simulink model "Simulacao_POSITIVO_LQG"  (R2020a)
settings: Solver=VariableStepAuto  StartTime=0.0  StopTime=15  RelTol=1e-6
values from neighbouring files (symbols this model uses):
  K1_rd1 = Kchz1(1,1)    [LQG_DIRSCRETO_1406_2025_NEGATIVO.m]    (also in LQG_DIRSCRETO_1406_2025_POSITIVO.m)
  K1_rd2 = Kchz2(1,1)    [LQG_DIRSCRETO_1406_2025_NEGATIVO.m]    (also in LQG_DIRSCRETO_1406_2025_POSITIVO.m)
  K1_rd3 = Kchz3(1,1)    [LQG_DIRSCRETO_1406_2025_NEGATIVO.m]    (also in LQG_DIRSCRETO_1406_2025_POSITIVO.m)
  K1_re1 = Kchz1(1,1)    [LQG_DIRSCRETO_1406_2025_NEGATIVO.m]    (also in LQG_DIRSCRETO_1406_2025_POSITIVO.m)
  K1_re2 = Kchz2(1,1)    [LQG_DIRSCRETO_1406_2025_NEGATIVO.m]    (also in LQG_DIRSCRETO_1406_2025_POSITIVO.m)
  K1_re3 = Kchz3(1,1)    [LQG_DIRSCRETO_1406_2025_NEGATIVO.m]    (also in LQG_DIRSCRETO_1406_2025_POSITIVO.m)
  Ki_rd1 = -Kchz1(1,2)    [LQG_DIRSCRETO_1406_2025_NEGATIVO.m]    (also in LQG_DIRSCRETO_1406_2025_POSITIVO.m)
  Ki_rd2 = -Kchz2(1,2)    [LQG_DIRSCRETO_1406_2025_NEGATIVO.m]    (also in LQG_DIRSCRETO_1406_2025_POSITIVO.m)
  Ki_rd3 = -Kchz3(1,2)    [LQG_DIRSCRETO_1406_2025_NEGATIVO.m]    (also in LQG_DIRSCRETO_1406_2025_POSITIVO.m)
  Ki_re1 = -Kchz1(1,2)    [LQG_DIRSCRETO_1406_2025_NEGATIVO.m]    (also in LQG_DIRSCRETO_1406_2025_POSITIVO.m)
  Ki_re2 = -Kchz2(1,2)    [LQG_DIRSCRETO_1406_2025_NEGATIVO.m]    (also in LQG_DIRSCRETO_1406_2025_POSITIVO.m)
  Ki_re3 = -Kchz3(1,2)    [LQG_DIRSCRETO_1406_2025_NEGATIVO.m]    (also in LQG_DIRSCRETO_1406_2025_POSITIVO.m)
  Ts = 0.02    [LQG_DIRSCRETO_1406_2025_NEGATIVO.m]    (also in LQG_DIRSCRETO_1406_2025_POSITIVO.m)
undefined symbols (not defined in the file or in its folder): A_rd1, A_rd2, A_rd3, A_re1, A_re2, A_re3, B_rd1, B_rd2, B_rd3, B_re1, B_re2, B_re3, C_rd1, C_rd2, C_rd3, C_re1, C_re2, C_re3, DiscIntNeverNeededParam, Ke_rd1, Ke_rd2, Ke_rd3, Ke_re1, Ke_re2, Ke_re3, sigbuilder_block
settings Model: Creator=vinic  LastModifiedBy=vinic

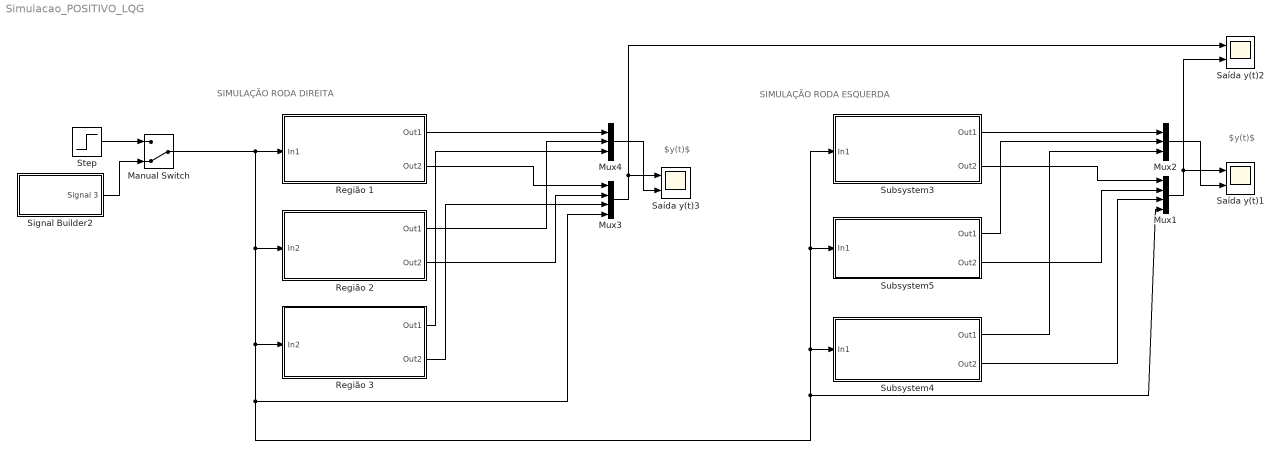
== system Simulacao_POSITIVO_LQG ==
  note: SIMULAÇÃO RODA ESQUERDA
  note: SIMULAÇÃO RODA DIREITA
  note: $y(t)$
  note: $y(t)$
  Manual Switch : ManualSwitch  CurrentSetting=0
  Mux1 : Mux
  Mux2 : Mux  Inputs=3
  Mux3 : Mux
  Mux4 : Mux  Inputs=3
  Região 1 : Subsystem
  Região 2 : Subsystem
  Região 3 : Subsystem
  Saída y(t)1 : Scope  NumInputPorts=2
  Saída y(t)2 : Scope  NumInputPorts=2
  Saída y(t)3 : Scope  NumInputPorts=2
  Signal Builder2 : Subsystem  Tag=STV Subsys  LoadFcn=sigbuilder_block('load');  StartFcn=sigbuilder_block('start');  StopFcn=sigbuilder_block('stop');  ClipboardFcn=sigbuilder_block('clipboard');  mask(Sigbuilder block){tuvar=[0:10]}
      mask help: Simulink:masks:SigbuilderBlock_MD
      mask init:
      | if ~strcmp(get_param(bdroot(gcbh),'SimulationStatus'),'stopped') tuvar = sigbuilder_block('maskInit'); end
      settings: CopyFcn=sigbuilder_block('copy');  DeleteFcn=sigbuilder_block('delete');  ModelCloseFcn=sigbuilder_block('modelClose');  PreSaveFcn=sigbuilder_block('preSave');  PauseFcn=sigbuilder_block('pause');  ContinueFcn=sigbuilder_block('continue');  NameChangeFcn=sigbuilder_block('namechange');  OpenFcn=sigbuilder_block('open',[5.4 36 1141.2 516.6 ]);  CloseFcn=sigbuilder_block('close');
      mask Display: plot(0, 0, 100, 100,[2, 2, 32, 32, 2], [68, 8, 8, 68, 68],[32, 2], [38, 38], [32, 19, 2],[53, 60, 44], [32, 17, 17, 2],[16, 16, 31, 31]);txt = getActiveGroup(gcbh);text(2, 100, txt,'verticalAlignment', 'top');
  Step : Step  Time=0  After=500  SampleTime=0.02
  Subsystem3 : Subsystem
  Subsystem4 : Subsystem
  Subsystem5 : Subsystem
  wires:
  Mux4/1 -> Saída y(t)3/2
  Step/1 -> Manual Switch/1
  Região 1/1(Out1) -> Mux4/1
  Região 2/1(Out1) -> Mux4/2
  Região 2/2(Out2) -> Mux3/2
  Região 3/1(Out1) -> Mux4/3
  Região 3/2(Out2) -> Mux3/3
  Mux3/1 -> Saída y(t)3/1, Saída y(t)2/1
  Região 1/2(Out2) -> Mux3/1
  Mux2/1 -> Saída y(t)1/2
  Subsystem5/2(Out2) -> Mux1/2
  Subsystem3/2(Out2) -> Mux1/1
  Subsystem5/1(Out1) -> Mux2/2
  Subsystem4/1(Out1) -> Mux2/3
  Mux1/1 -> Saída y(t)2/2, Saída y(t)1/1
  Subsystem4/2(Out2) -> Mux1/3
  Manual Switch/1 -> Região 3/1(In2), Mux3/4, Subsystem4/1(In1), Subsystem3/1(In1), Subsystem5/1(In1), Mux1/4, Região 2/1(In2), Região 1/1(In1)
  Subsystem3/1(Out1) -> Mux2/1
  Signal Builder2/1(Signal 3) -> Manual Switch/2

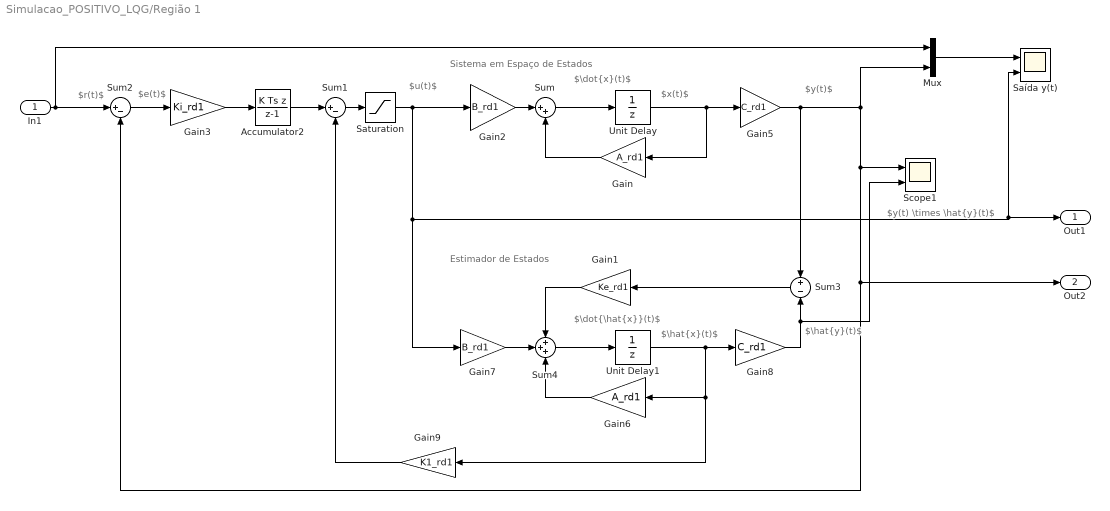
== system Simulacao_POSITIVO_LQG/Região 1 ==
  note: $\hat{y}(t)$
  note: Estimador de Estados
  note: $e(t)$
  note: $\dot{x}(t)$
  note: $\hat{x}(t)$
  note: $y(t)$
  note: $\dot{\hat{x}}(t)$
  note: $u(t)$
  note: $r(t)$
  note: $y(t) \times \hat{y}(t)$
  note: $x(t)$
  note: Sistema em Espaço de Estados
  In1 : Inport
  Accumulator2 : DiscreteIntegrator  IntegratorMethod=Integration: Backward Euler  SampleTime=Ts  ICPrevOutput=DiscIntNeverNeededParam  ICPrevScaledInput=DiscIntNeverNeededParam
  Gain : Gain  Gain=A_rd1
  Gain1 : Gain  Gain=Ke_rd1
  Gain2 : Gain  Gain=B_rd1
  Gain3 : Gain  Gain=Ki_rd1
  Gain5 : Gain  Gain=C_rd1
  Gain6 : Gain  Gain=A_rd1
  Gain7 : Gain  Gain=B_rd1
  Gain8 : Gain  Gain=C_rd1
  Gain9 : Gain  Gain=K1_rd1
  Mux : Mux  Inputs=2
  Saturation : Saturate  UpperLimit=100  LowerLimit=-100
  Saída y(t) : Scope  NumInputPorts=2
  Scope1 : Scope  NumInputPorts=2
  Sum : Sum  Inputs=|++
  Sum1 : Sum  Inputs=|+-
  Sum2 : Sum  Inputs=|+-
  Sum3 : Sum  Inputs=+|-
  Sum4 : Sum  Inputs=+++
  Unit Delay : UnitDelay  SampleTime=Ts  HasFrameUpgradeWarning=on
  Unit Delay1 : UnitDelay  SampleTime=Ts  HasFrameUpgradeWarning=on
  Out1 : Outport
  Out2 : Outport  Port=2
  wires:
  Mux/1 -> Saída y(t)/1
  Gain1/1 -> Sum4/1
  Gain6/1 -> Sum4/3
  Gain3/1 -> Accumulator2/1
  Saturation/1 -> Gain7/1, Out1/1, Saída y(t)/2, Gain2/1
  Sum1/1 -> Saturation/1
  Sum4/1 -> Unit Delay1/1
  Gain8/1 -> Scope1/2, Sum3/2
  Gain/1 -> Sum/2
  Unit Delay1/1 -> Gain9/1, Gain6/1, Gain8/1
  Gain5/1 -> Sum3/1, Scope1/1, Sum2/2, Out2/1, Mux/2
  Unit Delay/1 -> Gain5/1, Gain/1
  Gain9/1 -> Sum1/2
  Gain2/1 -> Sum/1
  Gain7/1 -> Sum4/2
  Sum2/1 -> Gain3/1
  Accumulator2/1 -> Sum1/1
  In1/1 -> Mux/1, Sum2/1
  Sum3/1 -> Gain1/1
  Sum/1 -> Unit Delay/1

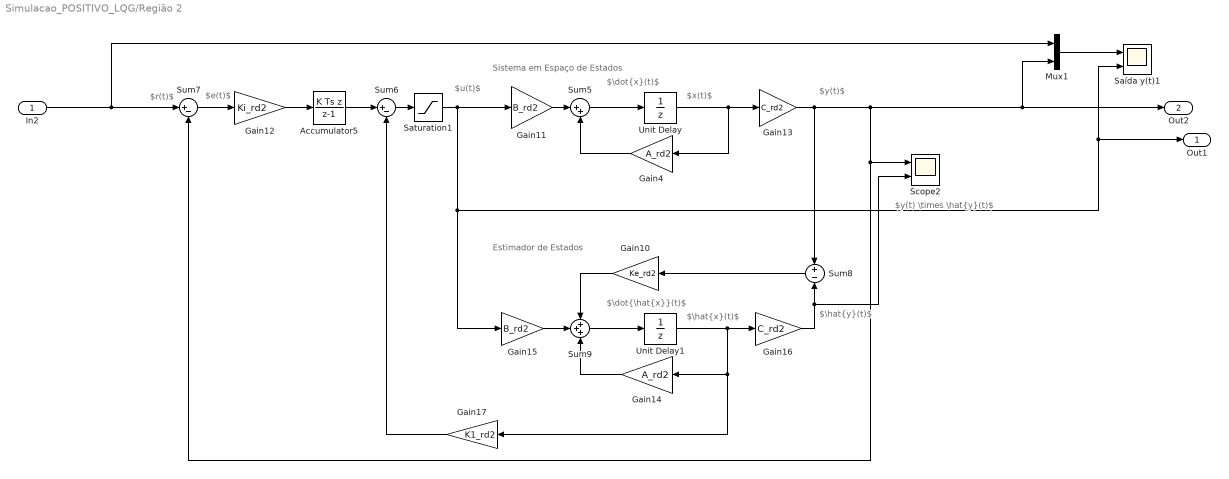
== system Simulacao_POSITIVO_LQG/Região 2 ==
  note: $r(t)$
  note: Sistema em Espaço de Estados
  note: $e(t)$
  note: $\dot{\hat{x}}(t)$
  note: $\hat{x}(t)$
  note: Estimador de Estados
  note: $x(t)$
  note: $u(t)$
  note: $y(t) \times \hat{y}(t)$
  note: $y(t)$
  note: $\hat{y}(t)$
  note: $\dot{x}(t)$
  In2 : Inport
  Accumulator5 : DiscreteIntegrator  IntegratorMethod=Integration: Backward Euler  SampleTime=Ts  ICPrevOutput=DiscIntNeverNeededParam  ICPrevScaledInput=DiscIntNeverNeededParam
  Gain10 : Gain  Gain=Ke_rd2
  Gain11 : Gain  Gain=B_rd2
  Gain12 : Gain  Gain=Ki_rd2
  Gain13 : Gain  Gain=C_rd2
  Gain14 : Gain  Gain=A_rd2
  Gain15 : Gain  Gain=B_rd2
  Gain16 : Gain  Gain=C_rd2
  Gain17 : Gain  Gain=K1_rd2
  Gain4 : Gain  Gain=A_rd2
  Mux1 : Mux  Inputs=2
  Saturation1 : Saturate  UpperLimit=100  LowerLimit=-100
  Saída y(t)1 : Scope  NumInputPorts=2
  Scope2 : Scope  NumInputPorts=2
  Sum5 : Sum  Inputs=|++
  Sum6 : Sum  Inputs=|+-
  Sum7 : Sum  Inputs=|+-
  Sum8 : Sum  Inputs=+|-
  Sum9 : Sum  Inputs=+++
  Unit Delay : UnitDelay  SampleTime=-1  HasFrameUpgradeWarning=on
  Unit Delay1 : UnitDelay  SampleTime=-1  HasFrameUpgradeWarning=on
  Out1 : Outport
  Out2 : Outport  Port=2
  wires:
  Gain13/1 -> Sum8/1, Mux1/2, Out2/1, Scope2/1, Sum7/2
  Gain10/1 -> Sum9/1
  Mux1/1 -> Saída y(t)1/1
  Unit Delay1/1 -> Gain17/1, Gain14/1, Gain16/1
  Sum9/1 -> Unit Delay1/1
  Gain15/1 -> Sum9/2
  Unit Delay/1 -> Gain13/1, Gain4/1
  Saturation1/1 -> Out1/1, Saída y(t)1/2, Gain15/1, Gain11/1
  Gain11/1 -> Sum5/1
  Gain17/1 -> Sum6/2
  Sum6/1 -> Saturation1/1
  Sum5/1 -> Unit Delay/1
  Gain16/1 -> Scope2/2, Sum8/2
  Accumulator5/1 -> Sum6/1
  Gain4/1 -> Sum5/2
  Gain12/1 -> Accumulator5/1
  Sum7/1 -> Gain12/1
  Gain14/1 -> Sum9/3
  In2/1 -> Mux1/1, Sum7/1
  Sum8/1 -> Gain10/1

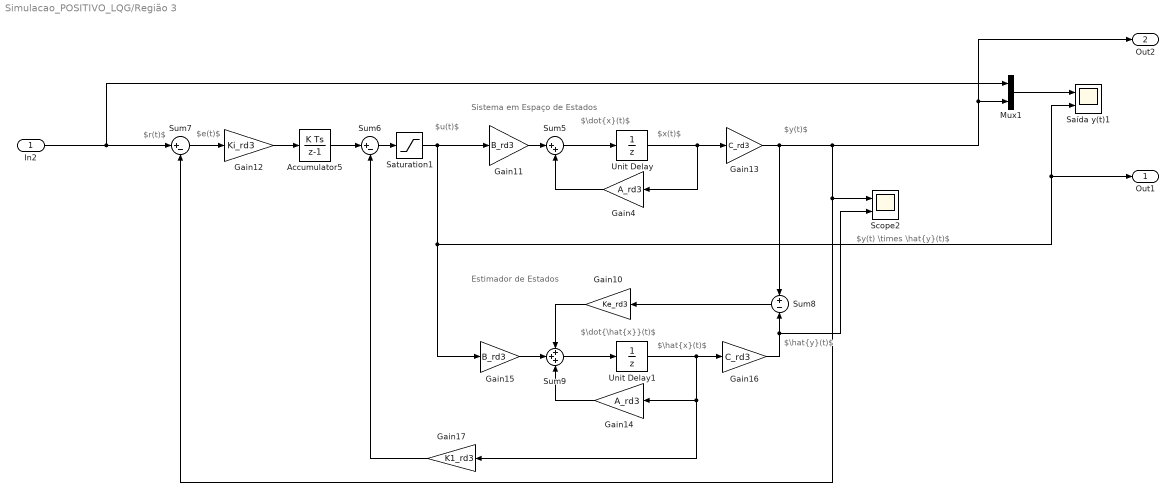
== system Simulacao_POSITIVO_LQG/Região 3 ==
  note: $\dot{\hat{x}}(t)$
  note: Estimador de Estados
  note: $y(t)$
  note: Sistema em Espaço de Estados
  note: $u(t)$
  note: $x(t)$
  note: $r(t)$
  note: $y(t) \times \hat{y}(t)$
  note: $e(t)$
  note: $\hat{y}(t)$
  note: $\dot{x}(t)$
  note: $\hat{x}(t)$
  In2 : Inport
  Accumulator5 : DiscreteIntegrator  SampleTime=Ts  ICPrevOutput=DiscIntNeverNeededParam  ICPrevScaledInput=DiscIntNeverNeededParam
  Gain10 : Gain  Gain=Ke_rd3
  Gain11 : Gain  Gain=B_rd3
  Gain12 : Gain  Gain=Ki_rd3
  Gain13 : Gain  Gain=C_rd3
  Gain14 : Gain  Gain=A_rd3
  Gain15 : Gain  Gain=B_rd3
  Gain16 : Gain  Gain=C_rd3
  Gain17 : Gain  Gain=K1_rd3
  Gain4 : Gain  Gain=A_rd3
  Mux1 : Mux  Inputs=2
  Saturation1 : Saturate  UpperLimit=100  LowerLimit=-100
  Saída y(t)1 : Scope  NumInputPorts=2
  Scope2 : Scope  NumInputPorts=2
  Sum5 : Sum  Inputs=|++
  Sum6 : Sum  Inputs=|+-
  Sum7 : Sum  Inputs=|+-
  Sum8 : Sum  Inputs=+|-
  Sum9 : Sum  Inputs=+++
  Unit Delay : UnitDelay  SampleTime=Ts  HasFrameUpgradeWarning=on
  Unit Delay1 : UnitDelay  SampleTime=Ts  HasFrameUpgradeWarning=on
  Out1 : Outport
  Out2 : Outport  Port=2
  wires:
  Unit Delay/1 -> Gain13/1, Gain4/1
  In2/1 -> Mux1/1, Sum7/1
  Gain14/1 -> Sum9/3
  Gain11/1 -> Sum5/1
  Gain12/1 -> Accumulator5/1
  Accumulator5/1 -> Sum6/1
  Sum7/1 -> Gain12/1
  Gain16/1 -> Scope2/2, Sum8/2
  Gain17/1 -> Sum6/2
  Saturation1/1 -> Out1/1, Saída y(t)1/2, Gain15/1, Gain11/1
  Unit Delay1/1 -> Gain17/1, Gain14/1, Gain16/1
  Gain15/1 -> Sum9/2
  Sum6/1 -> Saturation1/1
  Gain4/1 -> Sum5/2
  Gain13/1 -> Sum8/1, Mux1/2, Out2/1, Scope2/1, Sum7/2
  Sum5/1 -> Unit Delay/1
  Mux1/1 -> Saída y(t)1/1
  Gain10/1 -> Sum9/1
  Sum9/1 -> Unit Delay1/1
  Sum8/1 -> Gain10/1

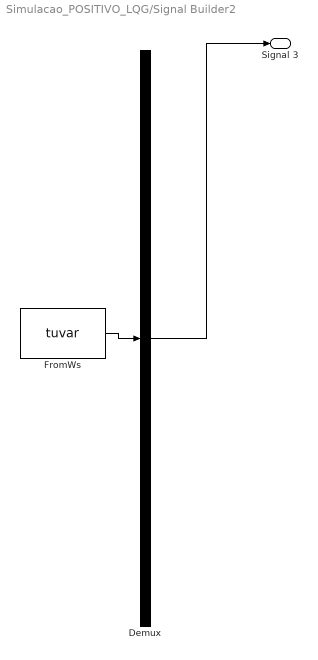
== system Simulacao_POSITIVO_LQG/Signal Builder2 ==
  Demux : Demux  Tag=STV Demux  Outputs=1
      settings: DisplayOption=none
  FromWs : FromWorkspace  Tag=STV FromWs  VariableName=tuvar
      SigBuilderData=|
      | common.afterFinalStr = 'Extrapolate'
      | common.sampleTime = 0
      | dataSet.timeRange = [0 15]
      | dataSet.name = 'Group 1'
      | sbobj.Groups.Name = 'Group 1'
      | sbobj.Groups.Signals.Name = 'Signal 3'
      | sbobj.Groups.Signals.XData = [0 2.5 2.5 5 5 7.5 7.5 10 10 12.5 12.5 15]
      | sbobj.Groups.Signals.YData = [320 320 560 560 800 800 400 400 640 640 480 480]
      | sbobj.Groups.TimeRange = [0 15]
  Signal 3 : Outport  Tag=STV Outport
  wires:
  FromWs/1 -> Demux/1
  Demux/1 -> Signal 3/1

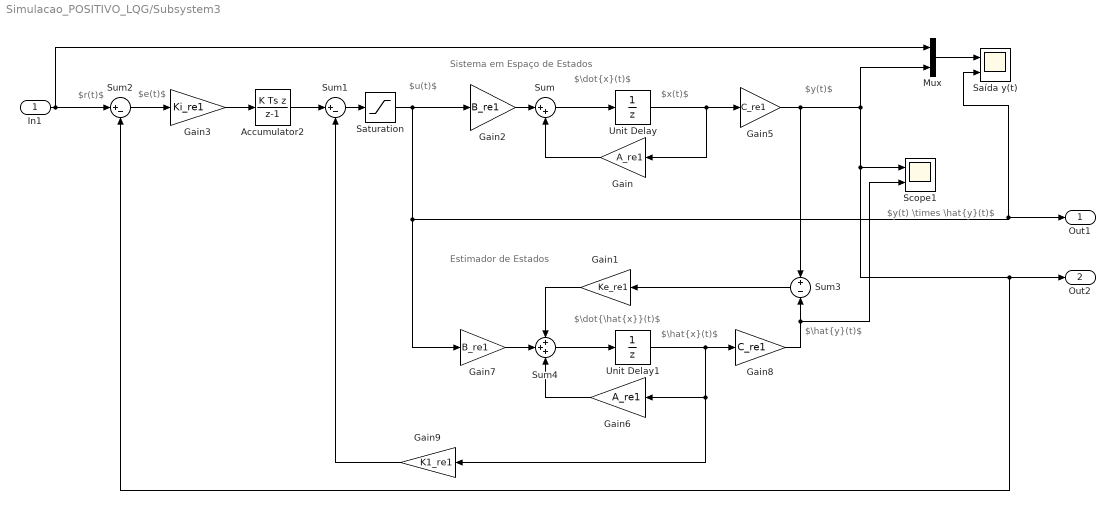
== system Simulacao_POSITIVO_LQG/Subsystem3 ==
  note: $\hat{y}(t)$
  note: Estimador de Estados
  note: $e(t)$
  note: $\dot{x}(t)$
  note: $\hat{x}(t)$
  note: $y(t)$
  note: $\dot{\hat{x}}(t)$
  note: $u(t)$
  note: $r(t)$
  note: $y(t) \times \hat{y}(t)$
  note: $x(t)$
  note: Sistema em Espaço de Estados
  In1 : Inport
  Accumulator2 : DiscreteIntegrator  IntegratorMethod=Integration: Backward Euler  SampleTime=Ts  ICPrevOutput=DiscIntNeverNeededParam  ICPrevScaledInput=DiscIntNeverNeededParam
  Gain : Gain  Gain=A_re1
  Gain1 : Gain  Gain=Ke_re1
  Gain2 : Gain  Gain=B_re1
  Gain3 : Gain  Gain=Ki_re1
  Gain5 : Gain  Gain=C_re1
  Gain6 : Gain  Gain=A_re1
  Gain7 : Gain  Gain=B_re1
  Gain8 : Gain  Gain=C_re1
  Gain9 : Gain  Gain=K1_re1
  Mux : Mux  Inputs=2
  Saturation : Saturate  UpperLimit=100  LowerLimit=-100
  Saída y(t) : Scope  NumInputPorts=2
  Scope1 : Scope  NumInputPorts=2
  Sum : Sum  Inputs=|++
  Sum1 : Sum  Inputs=|+-
  Sum2 : Sum  Inputs=|+-
  Sum3 : Sum  Inputs=+|-
  Sum4 : Sum  Inputs=+++
  Unit Delay : UnitDelay  SampleTime=Ts  HasFrameUpgradeWarning=on
  Unit Delay1 : UnitDelay  SampleTime=Ts  HasFrameUpgradeWarning=on
  Out1 : Outport
  Out2 : Outport  Port=2
  wires:
  Mux/1 -> Saída y(t)/1
  Gain1/1 -> Sum4/1
  Gain6/1 -> Sum4/3
  Gain3/1 -> Accumulator2/1
  Saturation/1 -> Gain7/1, Out1/1, Saída y(t)/2, Gain2/1
  Sum1/1 -> Saturation/1
  Sum4/1 -> Unit Delay1/1
  Gain8/1 -> Scope1/2, Sum3/2
  Gain/1 -> Sum/2
  Unit Delay1/1 -> Gain9/1, Gain6/1, Gain8/1
  Gain5/1 -> Sum3/1, Scope1/1, Sum2/2, Out2/1, Mux/2
  Unit Delay/1 -> Gain5/1, Gain/1
  Gain9/1 -> Sum1/2
  Gain2/1 -> Sum/1
  Gain7/1 -> Sum4/2
  Sum2/1 -> Gain3/1
  Accumulator2/1 -> Sum1/1
  In1/1 -> Mux/1, Sum2/1
  Sum3/1 -> Gain1/1
  Sum/1 -> Unit Delay/1

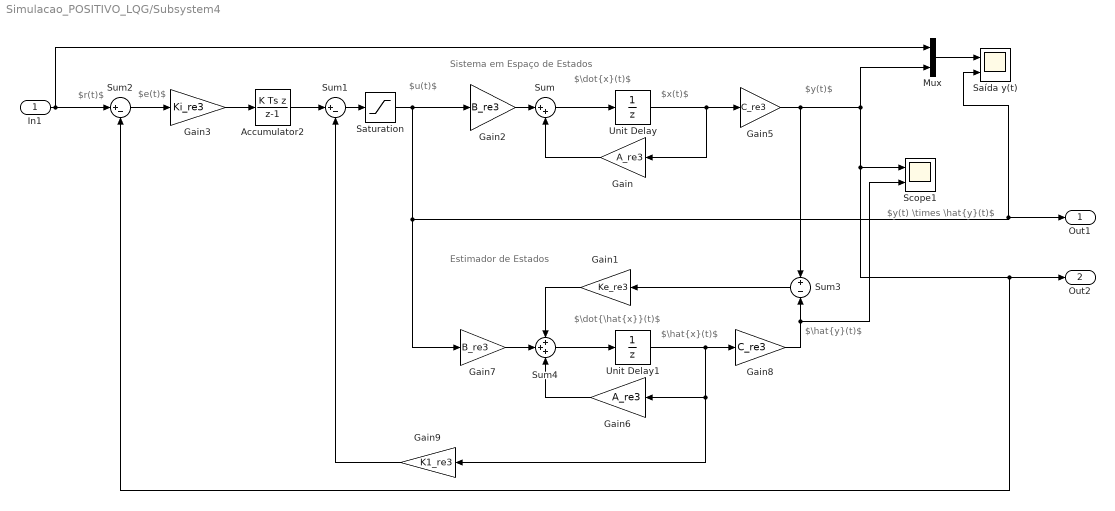
== system Simulacao_POSITIVO_LQG/Subsystem4 ==
  note: Estimador de Estados
  note: $e(t)$
  note: $\hat{y}(t)$
  note: $\dot{x}(t)$
  note: $y(t)$
  note: $u(t)$
  note: $r(t)$
  note: $\dot{\hat{x}}(t)$
  note: $x(t)$
  note: $y(t) \times \hat{y}(t)$
  note: $\hat{x}(t)$
  note: Sistema em Espaço de Estados
  In1 : Inport
  Accumulator2 : DiscreteIntegrator  IntegratorMethod=Integration: Backward Euler  SampleTime=Ts  ICPrevOutput=DiscIntNeverNeededParam  ICPrevScaledInput=DiscIntNeverNeededParam
  Gain : Gain  Gain=A_re3
  Gain1 : Gain  Gain=Ke_re3
  Gain2 : Gain  Gain=B_re3
  Gain3 : Gain  Gain=Ki_re3
  Gain5 : Gain  Gain=C_re3
  Gain6 : Gain  Gain=A_re3
  Gain7 : Gain  Gain=B_re3
  Gain8 : Gain  Gain=C_re3
  Gain9 : Gain  Gain=K1_re3
  Mux : Mux  Inputs=2
  Saturation : Saturate  UpperLimit=100  LowerLimit=-100
  Saída y(t) : Scope  NumInputPorts=2
  Scope1 : Scope  NumInputPorts=2
  Sum : Sum  Inputs=|++
  Sum1 : Sum  Inputs=|+-
  Sum2 : Sum  Inputs=|+-
  Sum3 : Sum  Inputs=+|-
  Sum4 : Sum  Inputs=+++
  Unit Delay : UnitDelay  SampleTime=Ts  HasFrameUpgradeWarning=on
  Unit Delay1 : UnitDelay  SampleTime=Ts  HasFrameUpgradeWarning=on
  Out1 : Outport
  Out2 : Outport  Port=2
  wires:
  Sum/1 -> Unit Delay/1
  Sum2/1 -> Gain3/1
  Sum3/1 -> Gain1/1
  Gain5/1 -> Sum3/1, Scope1/1, Sum2/2, Out2/1, Mux/2
  Accumulator2/1 -> Sum1/1
  Gain/1 -> Sum/2
  In1/1 -> Mux/1, Sum2/1
  Gain8/1 -> Scope1/2, Sum3/2
  Unit Delay1/1 -> Gain9/1, Gain6/1, Gain8/1
  Gain9/1 -> Sum1/2
  Gain1/1 -> Sum4/1
  Gain3/1 -> Accumulator2/1
  Gain2/1 -> Sum/1
  Saturation/1 -> Gain7/1, Out1/1, Saída y(t)/2, Gain2/1
  Gain7/1 -> Sum4/2
  Mux/1 -> Saída y(t)/1
  Sum1/1 -> Saturation/1
  Sum4/1 -> Unit Delay1/1
  Gain6/1 -> Sum4/3
  Unit Delay/1 -> Gain5/1, Gain/1

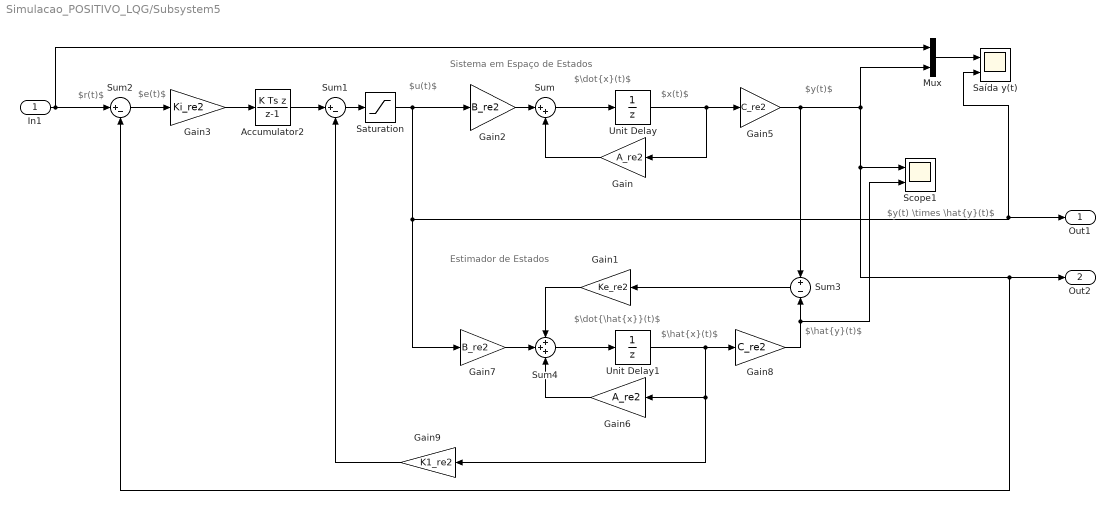
== system Simulacao_POSITIVO_LQG/Subsystem5 ==
  note: Estimador de Estados
  note: $e(t)$
  note: $\hat{y}(t)$
  note: $\dot{x}(t)$
  note: $y(t)$
  note: $u(t)$
  note: $r(t)$
  note: $\dot{\hat{x}}(t)$
  note: $x(t)$
  note: $y(t) \times \hat{y}(t)$
  note: $\hat{x}(t)$
  note: Sistema em Espaço de Estados
  In1 : Inport
  Accumulator2 : DiscreteIntegrator  IntegratorMethod=Integration: Backward Euler  SampleTime=Ts  ICPrevOutput=DiscIntNeverNeededParam  ICPrevScaledInput=DiscIntNeverNeededParam
  Gain : Gain  Gain=A_re2
  Gain1 : Gain  Gain=Ke_re2
  Gain2 : Gain  Gain=B_re2
  Gain3 : Gain  Gain=Ki_re2
  Gain5 : Gain  Gain=C_re2
  Gain6 : Gain  Gain=A_re2
  Gain7 : Gain  Gain=B_re2
  Gain8 : Gain  Gain=C_re2
  Gain9 : Gain  Gain=K1_re2
  Mux : Mux  Inputs=2
  Saturation : Saturate  UpperLimit=100  LowerLimit=-100
  Saída y(t) : Scope  NumInputPorts=2
  Scope1 : Scope  NumInputPorts=2
  Sum : Sum  Inputs=|++
  Sum1 : Sum  Inputs=|+-
  Sum2 : Sum  Inputs=|+-
  Sum3 : Sum  Inputs=+|-
  Sum4 : Sum  Inputs=+++
  Unit Delay : UnitDelay  SampleTime=Ts  HasFrameUpgradeWarning=on
  Unit Delay1 : UnitDelay  SampleTime=Ts  HasFrameUpgradeWarning=on
  Out1 : Outport
  Out2 : Outport  Port=2
  wires:
  Sum/1 -> Unit Delay/1
  Sum2/1 -> Gain3/1
  Sum3/1 -> Gain1/1
  Gain5/1 -> Sum3/1, Scope1/1, Sum2/2, Out2/1, Mux/2
  Accumulator2/1 -> Sum1/1
  Gain/1 -> Sum/2
  In1/1 -> Mux/1, Sum2/1
  Gain8/1 -> Scope1/2, Sum3/2
  Unit Delay1/1 -> Gain9/1, Gain6/1, Gain8/1
  Gain9/1 -> Sum1/2
  Gain1/1 -> Sum4/1
  Gain3/1 -> Accumulator2/1
  Gain2/1 -> Sum/1
  Saturation/1 -> Gain7/1, Out1/1, Saída y(t)/2, Gain2/1
  Gain7/1 -> Sum4/2
  Mux/1 -> Saída y(t)/1
  Sum1/1 -> Saturation/1
  Sum4/1 -> Unit Delay1/1
  Gain6/1 -> Sum4/3
  Unit Delay/1 -> Gain5/1, Gain/1
